simulink model "Buck_Type3compmodel"  (R2021a)
settings: Solver=VariableStepAuto  StartTime=0.0  StopTime=0.1  RelTol=1e-3
libraries: spsSeriesRLCBranchLib x7, spsVoltageMeasurementLib x3, spsCurrentMeasurementLib x2, spsDCVoltageSourceLib x1, spsDiodeLib x1, spsACVoltageSourceLib x1, spsGroundLib x1, spsMosfetLib x1, simulink x1, spspowerguiLib x1
settings Model: Creator=Lenovo  LastModifiedBy=Lenovo

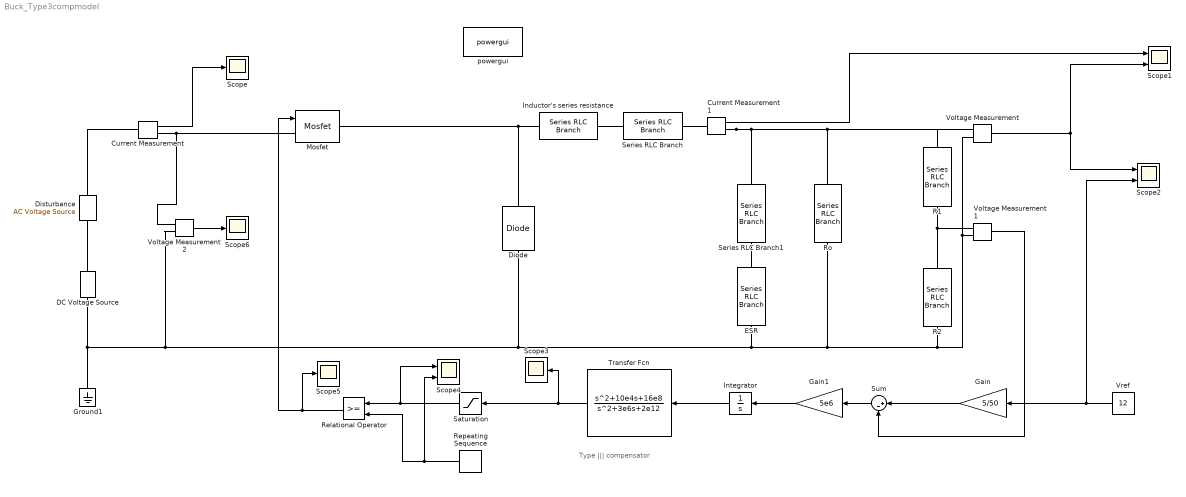
== system Buck_Type3compmodel ==
  note: Type ||| compensator
  Current Measurement : spsCurrentMeasurementLib/Current Measurement  PhasorSimulation=off  OutputType=Complex  PSBequivalent=0
  Current Measurement1 : spsCurrentMeasurementLib/Current Measurement  PhasorSimulation=off  OutputType=Complex  PSBequivalent=0
  DC Voltage Source : spsDCVoltageSourceLib/DC Voltage Source  Amplitude=48  Measurements=None
  Diode : spsDiodeLib/Diode  Ron=0.001  Lon=0  Vf=0.8  IC=0  UseSnubber=0  Rs=500  Cs=250e-9  Measurements=off
  Disturbance : spsACVoltageSourceLib/AC Voltage Source  Amplitude=3  Phase=0  Frequency=100  SampleTime=0  Measurements=None  BusType=swing  Pref=10e3  Qref=0  Qmin=-inf  Qmax=+inf
  ESR : spsSeriesRLCBranchLib/Series RLC Branch  LConnTagsString=__new0  RConnTagsString=__new0  BranchType=R  Resistance=0.05  Inductance=0.5e-3  SetiL0=off  InitialCurrent=0  Capacitance=0.5e-6  Setx0=off  InitialVoltage=0  Measurements=None
  Gain : Gain  Gain=5/50
  Gain1 : Gain  Gain=5e6
  Ground1 : spsGroundLib/Ground  LConnTagsString=a
  Inductor's series resistance : spsSeriesRLCBranchLib/Series RLC Branch  LConnTagsString=__new0  RConnTagsString=__new0  BranchType=R  Resistance=0.05  Inductance=0.5e-3  SetiL0=off  InitialCurrent=0  Capacitance=0.5e-6  Setx0=off  InitialVoltage=0  Measurements=None
  Integrator : Integrator
  Mosfet : spsMosfetLib/Mosfet  Ron=0.1  Lon=0  Rd=0.01  Vfd=0  IC=0  Rs=1e5  Cs=inf  Measurements=off
  R1 : spsSeriesRLCBranchLib/Series RLC Branch  LConnTagsString=__new0  RConnTagsString=__new0  BranchType=R  Resistance=10e3  Inductance=0.5e-3  SetiL0=off  InitialCurrent=0  Capacitance=0.5e-6  Setx0=off  InitialVoltage=0  Measurements=None
  R2 : spsSeriesRLCBranchLib/Series RLC Branch  LConnTagsString=__new0  RConnTagsString=__new0  BranchType=R  Resistance=1.1e3  Inductance=0.5e-3  SetiL0=off  InitialCurrent=0  Capacitance=0.5e-6  Setx0=off  InitialVoltage=0  Measurements=None
  Relational Operator : RelationalOperator  OutDataTypeStr=boolean  RndMeth=Simplest
  Repeating Sequence : simulink/Sources/Repeating Sequence  rep_seq_t=[0 10e-6]  rep_seq_y=[0 1]
  Ro : spsSeriesRLCBranchLib/Series RLC Branch  LConnTagsString=__new0  RConnTagsString=__new0  BranchType=R  Resistance=6  Inductance=0.5e-3  SetiL0=off  InitialCurrent=0  Capacitance=0.5e-6  Setx0=off  InitialVoltage=0  Measurements=None
  Saturation : Saturate  UpperLimit=0.9  LowerLimit=0.1
  Scope{,3,5..6} (4 alike) : Scope
  Scope1 : Scope  NumInputPorts=2
  Scope2 : Scope  NumInputPorts=2
  Scope4 : Scope  NumInputPorts=2
  Series RLC Branch : spsSeriesRLCBranchLib/Series RLC Branch  LConnTagsString=__new0  RConnTagsString=__new0  BranchType=L  Resistance=1  Inductance=0.5e-3  SetiL0=off  InitialCurrent=0  Capacitance=0  Setx0=off  InitialVoltage=0  Measurements=None
  Series RLC Branch1 : spsSeriesRLCBranchLib/Series RLC Branch  LConnTagsString=__new0  RConnTagsString=__new0  BranchType=C  Resistance=1  Inductance=0.5e-3  SetiL0=off  InitialCurrent=0  Capacitance=0.5e-6  Setx0=off  InitialVoltage=0  Measurements=None
  Sum : Sum  Inputs=|+-
  Transfer Fcn : TransferFcn  Numerator=[1 10e4 16e8]  Denominator=[1 3e6 2e12]
  Voltage Measurement : spsVoltageMeasurementLib/Voltage Measurement  PhasorSimulation=off  OutputType=Complex  PSBequivalent=0
  Voltage Measurement1 : spsVoltageMeasurementLib/Voltage Measurement  PhasorSimulation=off  OutputType=Complex  PSBequivalent=0
  Voltage Measurement2 : spsVoltageMeasurementLib/Voltage Measurement  PhasorSimulation=off  OutputType=Complex  PSBequivalent=0
  Vref : Constant  Value=12
  powergui : spspowerguiLib/powergui  Priority=1  SimulationMode=Continuous  SampleTime=50e-6  frequency=60  Iterations=50  frequencyindice=0  Pbase=100e6  ErrMax=1e-4  UnitsV=kV  UnitsW=MW  buscounter=0  FunctionMessages=off  echomessages=off  EnableUseOfTLC=off  CurrentSourceSwitches=off  DisableSnubberDevices=off  DisableRonSwitches=off  DisableVfSwitches=off  DisplayEquations=off  AutomaticDiscreteSolvers=off  SolverType=Tustin/Backward Euler (TBE)  Interpol=off  ExternalGateDelay=off  methode=off  Ts=100  x0status=blocks  SPID=on  SwTol=0  HookPort=off  NonlinearTolerance=1e-4  nMaxIteration=100  ContinueOnMaxIteration=off  RestoreLinks=warning  ResistiveCurrentMeasurement=off  Frange=[0:2:500]  Ylog=off  Xlog=on  ShowGrid=off  save=off  variable=ZData  structure=0  ZoomFFT=off  StartTime=0.0  cycles=1  DisplayStyle=1  fundamental=60  FreqAxis=off  MaxFrequency=1000  frequencyindicesteady=1  RmsSteady=1  display=off
  wires:
  Current Measurement/1 -> Scope/1
  Current Measurement1/1 -> Scope1/1
  Voltage Measurement/1 -> Scope1/2, Scope2/1
  Vref/1 -> Scope2/2, Gain/1
  Gain/1 -> Sum/1
  Voltage Measurement1/1 -> Sum/2
  Sum/1 -> Gain1/1
  Gain1/1 -> Integrator/1
  Integrator/1 -> Transfer Fcn/1
  Transfer Fcn/1 -> Saturation/1, Scope3/1
  Saturation/1 -> Scope4/1, Relational Operator/1
  Repeating Sequence/1 -> Scope4/2, Relational Operator/2
  Relational Operator/1 -> Scope5/1, Mosfet/1
  Voltage Measurement2/1 -> Scope6/1
  connections:
  Mosfet/LConn1 -- Voltage Measurement2/LConn1 -- Current Measurement/RConn1
  Mosfet/RConn1 -- Diode/RConn1 -- Inductor's series resistance/RConn1
  Current Measurement1/LConn1 -- Series RLC Branch/RConn1
  R2/LConn1 -- Voltage Measurement1/LConn1 -- R1/RConn1
  Current Measurement1/RConn1 -- R1/LConn1 -- Voltage Measurement/LConn1 -- Ro/LConn1 -- Series RLC Branch1/LConn1
  Series RLC Branch1/RConn1 -- ESR/RConn1
  Current Measurement/LConn1 -- Disturbance/RConn1
  Disturbance/LConn1 -- DC Voltage Source/RConn1
  Inductor's series resistance/LConn1 -- Series RLC Branch/LConn1
  Voltage Measurement1/LConn2 -- R2/RConn1 -- Ro/RConn1 -- ESR/LConn1 -- Diode/LConn1 -- Voltage Measurement2/LConn2 -- Ground1/LConn1 -- DC Voltage Source/LConn1 -- Voltage Measurement/LConn2
